simulink model "simulink_GA_id"  (R2018b)
settings: Solver=VariableStepAuto  StartTime=0.0  StopTime=10.0  RelTol=1e-3
model workspace: external: MAT-File C:\Users\Emmanuel\Documents\MATLAB\script_GA_id_simulink.mat (data not in the file)
settings Model: Creator=Emmanuel  LastModifiedBy=Emmanuel

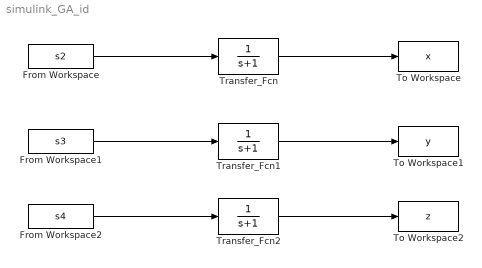
== system simulink_GA_id ==
  From Workspace : FromWorkspace  VariableName=s2  SampleTime=0
  From Workspace1 : FromWorkspace  VariableName=s3  SampleTime=0
  From Workspace2 : FromWorkspace  VariableName=s4  SampleTime=0
  To Workspace : ToWorkspace  VariableName=x  SampleTime=-1
  To Workspace1 : ToWorkspace  VariableName=y  SampleTime=-1
  To Workspace2 : ToWorkspace  VariableName=z  SampleTime=-1
  Transfer_Fcn : TransferFcn  Denominator=[1 1]
  Transfer_Fcn1 : TransferFcn  Denominator=[1 1]
  Transfer_Fcn2 : TransferFcn  Denominator=[1 1]
  wires:
  From Workspace/1 -> Transfer_Fcn/1
  Transfer_Fcn/1 -> To Workspace/1
  From Workspace1/1 -> Transfer_Fcn1/1
  Transfer_Fcn1/1 -> To Workspace1/1
  From Workspace2/1 -> Transfer_Fcn2/1
  Transfer_Fcn2/1 -> To Workspace2/1
